simulink model "Comparison-Karşılaştırma"  (R2024b)
settings: Solver=VariableStepAuto  StartTime=0.0  StopTime=10.0  MaxStep=0.01  RelTol=1e-3
settings Model: Creator=AliTeknik  LastModifiedBy=AliTeknik

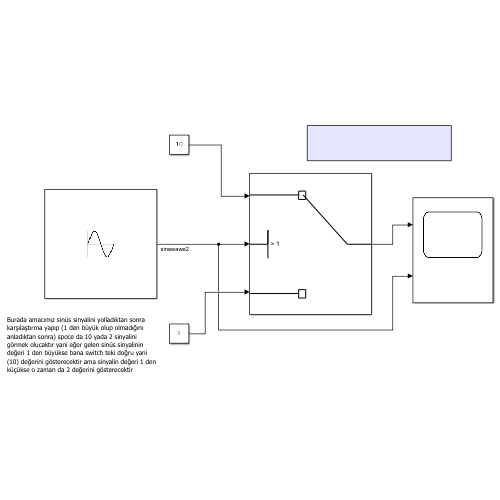
[thumbnail: Simulink's stored preview of the top-level diagram]
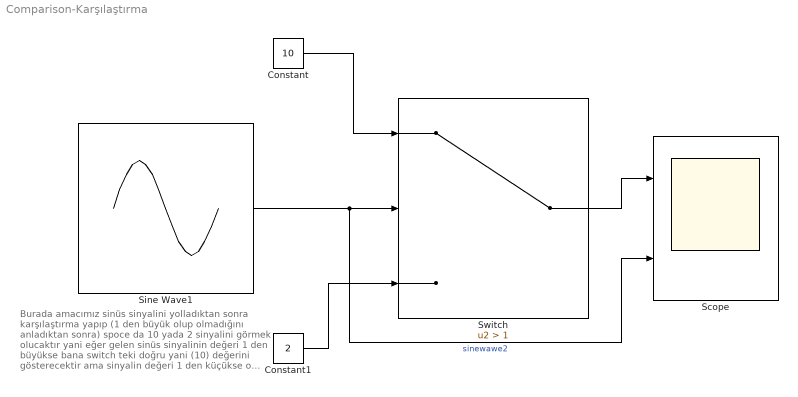
== system Comparison-Karşılaştırma ==
  note: Burada amacımız sinüs sinyalini yolladıktan sonra
      | karşılaştırma yapıp (1 den büyük olup olmadığını
      | anladıktan sonra) spoce da 10 yada 2 sinyalini
      | görmek olucaktır yani eğer gelen sinüs sinyalinin
      | değeri 1 den büyükse bana switch teki doğru yani
      | (10) değerini gösterecektir ama sinyalin değeri 1 den
      | küçükse o zaman da 2 değerini gösterecektir
  Constant : Constant  Value=10
  Constant1 : Constant  Value=2
  Scope : Scope  NumInputPorts=2
  Sine Wave1 : Sin  Amplitude=2  Frequency=5  SampleTime=0
  Switch : Switch  Criteria=u2 > Threshold  Threshold=1  SaturateOnIntegerOverflow=off  InputSameDT=off
  wires:
  Constant/1 -> Switch/1
  Constant1/1 -> Switch/3
  Sine Wave1/1 -> Scope/2, Switch/2  "sinewawe2"
  Switch/1 -> Scope/1
